simulink model "BBB_Compass_Test"  (R2013a)
settings: Solver=FixedStepDiscrete  StartTime=0.0  StopTime=inf  FixedStep=0.01  RelTol=1e-3
settings Model: SimulationMode=external  ExtModeTrigDuration=100  Creator=rdustinkahawita  LastModifiedBy=rdustinkahawita
settings OptimizationCC: OptimizeModelRefInitCode=on  LifeSpan=1
settings DebuggingCC: SolverPrmCheckMsg=none  StrictBusMsg=Warning
settings HardwareCC: ProdLargestAtomicInteger=Long  ProdLargestAtomicFloat=Double  ProdEndianess=LittleEndian  ProdHWDeviceType=ARM Compatible->ARM Cortex
settings RTWCC: SystemTargetFile=realtime.tlc  GenerateMakefile=off  TemplateMakefile=realtime.tmf  Description=Run on Target Hardware  RTWVerbose=off  ProcessScript=realtime_make_rtw_hook
settings STFCustomTargetCC: TargetLibSuffix=.a  GenerateSampleERTMain=on  ERTCustomFileBanners=on  SupportNonInlinedSFcns=off  SupportVariableSizeSignals=on  MATLABClassNameForMDSCustomization=Simulink.SoftwareTarget.ERTCustomization  SystemTargetFile=realtime.tlc
settings ERTTargetCC: ParMdlRefBuildCompliant=off  CompOptLevelCompliant=off  ConcurrentExecutionCompliant=off  CombineOutputUpdateFcns=off  ERTFirstTimeCompliant=off  SupportContinuousTime=on  SupportVariableSizeSignals=on  ModelStepFunctionPrototypeControlCompliant=off  CPPClassGenCompliant=off  ExtMode=on  ExtModeMexArgs='192.168.7.2' 0 17725  ERTSrcFileBannerTemplate=realtime_code_template.cgt  ERTHdrFileBannerTemplate=realtime_code_template.cgt  ERTDataSrcFileTemplate=realtime_code_template.cgt  ERTDataHdrFileTemplate=realtime_code_template.cgt  ERTCustomFileTemplate=realtime_file_process.tlc

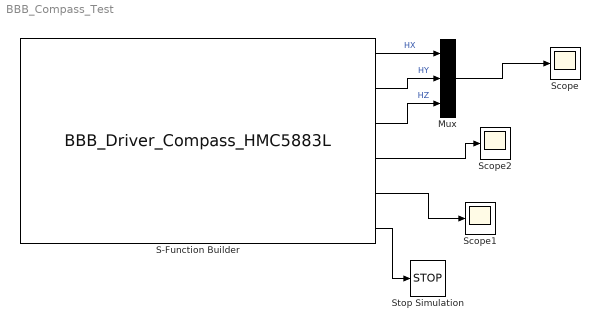
== system BBB_Compass_Test ==
  Mux : Mux  Inputs=3
  S-Function Builder : S-Function  InitFcn=try, set_param(gcb,'FunctionName','BBB_Driver_Compass_HMC5883L'), end  FunctionName=BBB_Driver_Compass_HMC5883L  Parameters=uint8(1),uint8(1),uint8(1),uint8(7),uint8(1),uint8(4),uint8(1),uint8(1),0.0,-14.66,boolean(1),uint8(6),uint8(7)  SFunctionModules=BBB_Driver_Compass_HMC5883L_wrapper  EnableBusSupport=off  mask(S-Function Builder){}
      mask help: Simulink:masks:SFunctionBuilder_MD
      mask init:
      | val = [[.9  0.75 0.75 1 1 .9 .9 1]',[1 1 0.75 0.75 .9 .9 1 .9]'];try , sys = get_param(gcb,'SfunBuilderFcnName');if isempty(sys), sys = get_param(gcb,'FunctionName'); end,catch, sys = get_param(gcb,'FunctionName'); end
      settings: CopyFcn=set_param(gcbh,'LinkStatus','none')  PreSaveFcn=try, set_param(gcb,'FunctionName','BBB_Driver_Compass_HMC5883L'), end  OpenFcn=sfunctionwizard(gcbh)
      mask Display: plot(val(:,1),val(:,2)),disp(sys), port_label('output',1,'outMagField_HX'), port_label('output',2,'outMagField_HY'), port_label('output',3,'outMagField_HZ'), port_label('output',4,'outMagField_HE'), port_label('output',5,'outMagField_Heading'), port_label('output',6,'outSimStop')
  Scope : Scope
      settings: ShowLegends=on  YMin=-35  YMax=55  SampleInput=on
  Scope1 : Scope
      settings: YMin=0  YMax=375
  Scope2 : Scope
      settings: YMin=40  YMax=48.5  SaveName=ScopeData2
  Stop Simulation : Stop
  wires:
  S-Function Builder/1 -> Mux/1  "HX"
  S-Function Builder/2 -> Mux/2  "HY"
  S-Function Builder/3 -> Mux/3  "HZ"
  Mux/1 -> Scope/1
  S-Function Builder/4 -> Scope2/1
  S-Function Builder/5 -> Scope1/1
  S-Function Builder/6 -> Stop Simulation/1
